simulink model "sampleModel77"  (R2021b)
settings: Solver=VariableStepAuto  StartTime=0.0  StopTime=10.0  RelTol=1e-3
undefined symbols (not defined in the file or in its folder): DiscIntNeverNeededParam
libraries: simulink x6
settings Model: Creator=user  LastModifiedBy=user

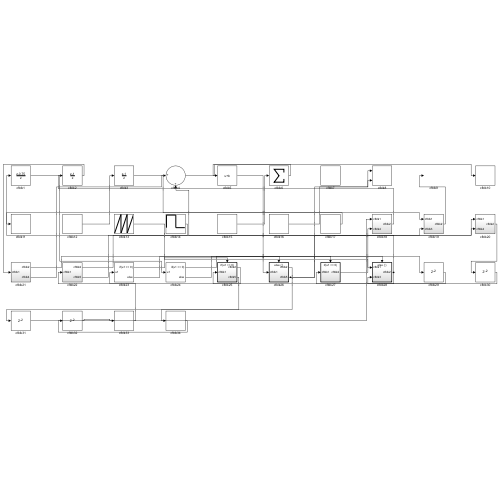
[thumbnail: Simulink's stored preview of the top-level diagram]
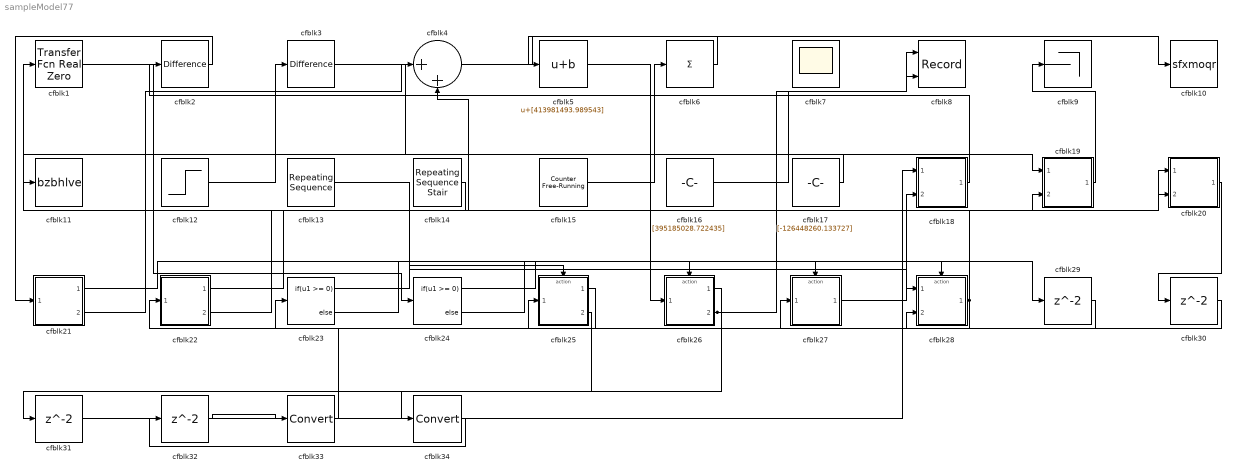
== system sampleModel77 ==
  cfblk1 : simulink/Discrete/Transfer Fcn Real Zero  ZeroZ=0.75  ICPrevInput=0.0  DoSatur=off
      settings: SourceProductBaseCode=SL
  cfblk10 : ToWorkspace  VariableName=sfxmoqr  SaveFormat=Timeseries  SampleTime=-1
  cfblk11 : ToWorkspace  VariableName=bzbhlve  SaveFormat=Timeseries  SampleTime=-1
  cfblk12 : Step  Time=[2.000000]  Before=[885551163.942840]  After=[-223459222.155460]  SampleTime=0
  cfblk13 : simulink/Sources/Repeating Sequence  rep_seq_t=[0 2]  rep_seq_y=[-735764767.115708, 650617970.515915]
  cfblk14 : simulink/Sources/Repeating Sequence Stair  OutValues=[715966432.186176, 537026367.980990]  tsamp=-1  OutMin=[]  OutMax=[]  OutDataTypeStr=double  OutputDataTypeScalingMode=double  OutDataType=fixdt(0,8)  ConRadixGroup=Best Precision: Vector-wise  OutScaling=2^-12
  cfblk15 : simulink/Sources/Counter Free-Running  NumBits=[53.000000]  tsamp=-1
  cfblk16 : Constant  Value=[395185028.722435]  SampleTime=1
  cfblk17 : Constant  Value=[-126448260.133727]  SampleTime=1
  cfblk18 : Subsystem
  cfblk19 : Subsystem
  cfblk2 : simulink/Discrete/Difference  ICPrevInput=0.0  OutMin=[]  OutMax=[]  OutDataTypeStr=Inherit: Inherit via back propagation  OutDataType=fixdt(1, 16)  OutScaling=2^-10  DoSatur=off
  cfblk20 : Subsystem
  cfblk21 : Subsystem
  cfblk22 : Subsystem
  cfblk23 : If  IfExpression=u1 >= 0  SampleTime=1
  cfblk24 : If  IfExpression=u1 >= 0  SampleTime=1
  cfblk25 : Subsystem  TreatAsAtomicUnit=on
  cfblk26 : Subsystem  TreatAsAtomicUnit=on
  cfblk27 : Subsystem  TreatAsAtomicUnit=on
  cfblk28 : Subsystem  TreatAsAtomicUnit=on
  cfblk{29..32} (4 alike) : Delay  SampleTime=1
  cfblk3 : simulink/Discrete/Difference  ICPrevInput=0.0  OutMin=[]  OutMax=[]  OutDataTypeStr=Inherit: Inherit via back propagation  OutDataType=fixdt(1, 16)  OutScaling=2^-10  DoSatur=off
  cfblk33 : DataTypeConversion
  cfblk34 : DataTypeConversion
  cfblk4 : Sum  Inputs=|++
  cfblk5 : Bias  Bias=[413981493.989543]
  cfblk6 : Sum  Inputs=+
  cfblk7 : Scope
      settings: Floating=on
  cfblk8 : Record  FileSettingsInternal="{\"entries\":[{\"content\":{\"excelSettings\":{\"content\":{},\"type\":\"Streamout.ExcelSettings\"}},\"type\":\"Streamout.FileSettingStorage\",\"uuid\":\"c65e012c-fb68-4e63-aaa4-e8d7c053a98a\"}],\"packageUris\":[\"http://schema.mathworks.com/mf0/streamout_blocks/R2020a\"],\"version\":\"1.0\"}"  Layout=[1 1]  SignalsInternal="{\"entries\":[{\"content\":{\"signals\":[{\"content\":{\"blockPath\":[\"sampleModel77/cfblk8\"],\"channel\":[],\"dimensions\":[1],\"domain\":\"sampleModel77/cfblk8\",\"lineColor\":\"#a2142f\",\"plots\":[1],\"port\":1,\"sid\":[\"\"],\"signalID\":2825,\"signalName\":\"cfblk16\"},\"type\":\"RecordBlkView.Signal\",\"uuid\":\"7f1cc23f-f652-48df-817a-9df80a368617\"},{\"content\":{\"blockPath\":[\"sampleModel77/cfblk8\"],\"channel\":[],\"dimensions\":[1],\"domain\":\"sampleModel77/cfblk8\",\"lineColor\":\"#139fff\",\"plots\":[1],\"port\":2,\"sid\":[\"\"],\"signalID\":2829,\"signalName\":\"cfblk26:2\"},\"type\":\"RecordBlkView.Signal\",\"uuid\":\"73d64d90-53f6-4771-93c0-51c4dd08edbd\"}]},\"type\":\"RecordBlkView.InputSignals\",\"uuid\":\"ea9197a5-161d-47c4-b8bf-a3b73525fcd2\"}],\"packageUris\":[\"http://schema.mathworks.com/mf0/streamout_blocks/R2020a\"],\"version\":\"1.0\"}"  VisualizationBindings="{\"xyplotplugin\":{\"info\":[{\"series\":[{\"bindingParametersList\":[{\"parameter\":\"X-Axis\",\"signalID\":2825,\"signalName\":\"cfblk16\"},{\"parameter\":\"Y-Axis\",\"signalID\":2829,\"signalName\":\"cfblk26:2\"}],\"seriesID\":10235}],\"subplotID\":1}]}}"  CompatibilityTag=XY
  cfblk9 : Terminator
  wires:
  cfblk3/1 -> cfblk19/1(cfblk1)
  cfblk14/1 -> cfblk1/1
  cfblk2/1 -> cfblk21/1(cfblk1)
  cfblk15/1 -> cfblk6/1
  cfblk4/1 -> cfblk10/1
  cfblk25/1(cfblk2) -> cfblk22/1(cfblk1)
  cfblk1/1 -> cfblk24/1
  cfblk18/1(cfblk2) -> cfblk2/1
  cfblk5/1 -> cfblk26/1(cfblk1)
  cfblk19/1(cfblk2) -> cfblk9/1
  cfblk28/1(cfblk2) -> cfblk25/1(cfblk1), cfblk4/2
  cfblk17/1 -> cfblk11/1
  cfblk27/1(cfblk2) -> cfblk18/2(cfblk4)
  cfblk12/1 -> cfblk3/1
  cfblk22/1(cfblk2) -> cfblk20/1(cfblk1)
  cfblk22/2(cfblk5) -> cfblk20/2(cfblk4)
  cfblk6/1 -> cfblk5/1
  cfblk13/1 -> cfblk28/1(cfblk1)
  cfblk21/2(cfblk4) -> cfblk4/1
  cfblk16/1 -> cfblk8/1
  cfblk26/2(cfblk5) -> cfblk8/2, cfblk19/2(cfblk3)
  cfblk23/1 -> cfblk25/Action
  cfblk23/2 -> cfblk26/Action
  cfblk24/1 -> cfblk27/Action
  cfblk24/2 -> cfblk28/Action
  cfblk21/1(cfblk2) -> cfblk29/1
  cfblk29/1 -> cfblk28/2(cfblk3)
  cfblk20/1(cfblk2) -> cfblk30/1
  cfblk30/1 -> cfblk27/1(cfblk1)
  cfblk25/2(cfblk5) -> cfblk31/1
  cfblk31/1 -> cfblk18/1(cfblk1)
  cfblk32/1 -> cfblk33/1
  cfblk33/1 -> cfblk23/1
  cfblk26/1(cfblk2) -> cfblk34/1
  cfblk34/1 -> cfblk32/1

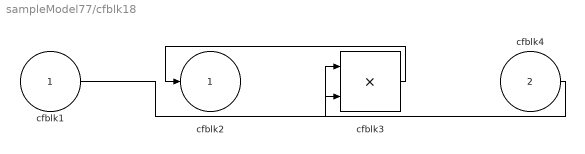
== system sampleModel77/cfblk18 ==
  cfblk1 : Inport
  cfblk4 : Inport  Port=2
  cfblk3 : Product
  cfblk2 : Outport
  wires:
  cfblk3/1 -> cfblk2/1
  cfblk1/1 -> cfblk3/1
  cfblk4/1 -> cfblk3/2

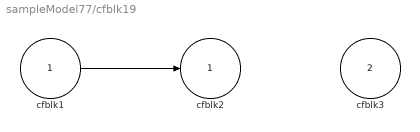
== system sampleModel77/cfblk19 ==
  cfblk1 : Inport
  cfblk3 : Inport  Port=2
  cfblk2 : Outport
  wires:
  cfblk1/1 -> cfblk2/1

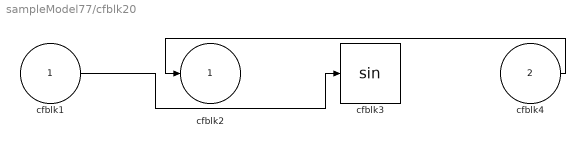
== system sampleModel77/cfblk20 ==
  cfblk1 : Inport
  cfblk4 : Inport  Port=2
  cfblk3 : Trigonometry
  cfblk2 : Outport
  wires:
  cfblk4/1 -> cfblk2/1
  cfblk1/1 -> cfblk3/1

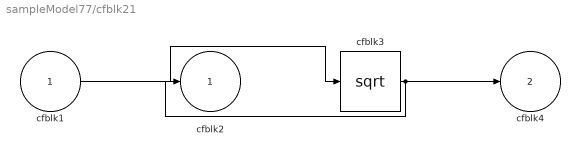
== system sampleModel77/cfblk21 ==
  cfblk1 : Inport
  cfblk3 : Sqrt  SaturateOnIntegerOverflow=on
  cfblk2 : Outport
  cfblk4 : Outport  Port=2
  wires:
  cfblk1/1 -> cfblk3/1
  cfblk3/1 -> cfblk2/1, cfblk4/1

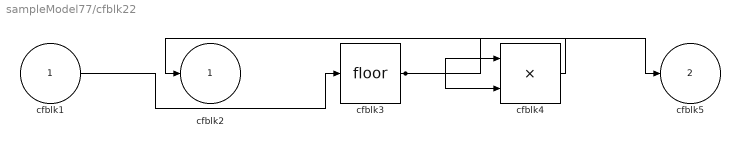
== system sampleModel77/cfblk22 ==
  cfblk1 : Inport
  cfblk3 : Rounding
  cfblk4 : Product  Inputs=**
  cfblk2 : Outport
  cfblk5 : Outport  Port=2
  wires:
  cfblk4/1 -> cfblk2/1
  cfblk1/1 -> cfblk3/1
  cfblk3/1 -> cfblk4/1, cfblk4/2, cfblk5/1

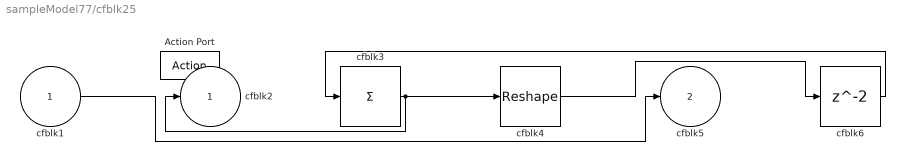
== system sampleModel77/cfblk25 ==
  cfblk1 : Inport
  Action Port : ActionPort  ActionPortLabel=if(u1 >= 0)
  cfblk3 : Sum  Inputs=+
  cfblk4 : Reshape
  cfblk6 : Delay
  cfblk2 : Outport
  cfblk5 : Outport  Port=2
  wires:
  cfblk3/1 -> cfblk2/1, cfblk4/1
  cfblk1/1 -> cfblk5/1
  cfblk4/1 -> cfblk6/1
  cfblk6/1 -> cfblk3/1

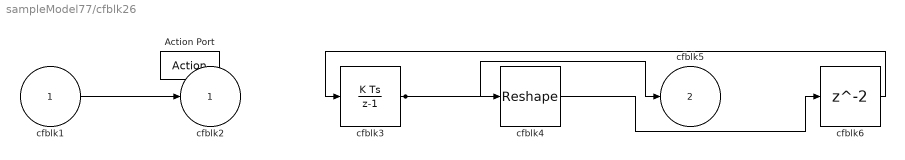
== system sampleModel77/cfblk26 ==
  cfblk1 : Inport
  Action Port : ActionPort  ActionPortLabel=else
  cfblk3 : DiscreteIntegrator  SampleTime=-1  ICPrevOutput=DiscIntNeverNeededParam  ICPrevScaledInput=DiscIntNeverNeededParam
  cfblk4 : Reshape
  cfblk6 : Delay
  cfblk2 : Outport
  cfblk5 : Outport  Port=2
  wires:
  cfblk1/1 -> cfblk2/1
  cfblk3/1 -> cfblk4/1, cfblk5/1
  cfblk4/1 -> cfblk6/1
  cfblk6/1 -> cfblk3/1

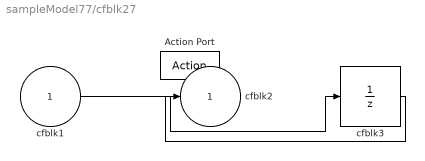
== system sampleModel77/cfblk27 ==
  cfblk1 : Inport
  Action Port : ActionPort  ActionPortLabel=if(u1 >= 0)
  cfblk3 : UnitDelay  SampleTime=-1  HasFrameUpgradeWarning=on
  cfblk2 : Outport
  wires:
  cfblk1/1 -> cfblk3/1
  cfblk3/1 -> cfblk2/1

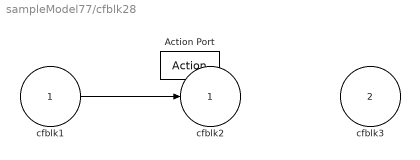
== system sampleModel77/cfblk28 ==
  cfblk1 : Inport
  cfblk3 : Inport  Port=2
  Action Port : ActionPort  ActionPortLabel=else
  cfblk2 : Outport
  wires:
  cfblk1/1 -> cfblk2/1
